simulink model "Zmixed_new"  (R2020b)
settings: Solver=FixedStepAuto  StartTime=0.0  StopTime=80000  FixedStep=1  RelTol=1e-3
values from neighbouring files (symbols this model uses):
  Inputp2 = data(1:IT,12)    [MainRun_step1__LoadData_and_DefineVaribles.m]
  InputT1 = data(1:IT,13)    [MainRun_step1__LoadData_and_DefineVaribles.m]
  InputWP = data(1:IT,66)    [MainRun_step1__LoadData_and_DefineVaribles.m]
  InputWT = data(1:IT,67)    [MainRun_step1__LoadData_and_DefineVaribles.m]
  Lp1 = data(1:IT,56)    [MainRun_step1__LoadData_and_DefineVaribles.m]
  Lp2 = data(1:IT,57)    [MainRun_step1__LoadData_and_DefineVaribles.m]
  T1 = data(1:IT,14)    [MainRun_step1__LoadData_and_DefineVaribles.m]
  Tamb = data(1:IT,55)    [MainRun_step1__LoadData_and_DefineVaribles.m]
  Tf1 = data(1:IT,16)    [MainRun_step1__LoadData_and_DefineVaribles.m]
  Tg1 = data(1:IT,53)    [MainRun_step1__LoadData_and_DefineVaribles.m]
  Tm = mean(data(1:IT,23:38),2)    [MainRun_step1__LoadData_and_DefineVaribles.m]
  WG = data(1:IT,51)    [MainRun_step1__LoadData_and_DefineVaribles.m]
  WR = data(1:IT,52)    [MainRun_step1__LoadData_and_DefineVaribles.m]
  Wtf = data(1:IT,15)    [MainRun_step1__LoadData_and_DefineVaribles.m]
  x = data(1:IT,49)    [MainRun_step1__LoadData_and_DefineVaribles.m]
  Zf = data(1:IT,50)    [MainRun_step1__LoadData_and_DefineVaribles.m]
undefined symbols (not defined in the file or in its folder): get_hs, precl, preclcp, precllamda, preclP, preclPP, preclT, refpropV
settings Model: Creator=Y7000  LastModifiedBy=admin
settings DataIOCC: ReturnWorkspaceOutputs=off
settings DebuggingCC: ArithmeticOperatorsInVariantConditions=warning
settings SFSimCC: CustomCodeUndefinedFunction=UseInterfaceOnly

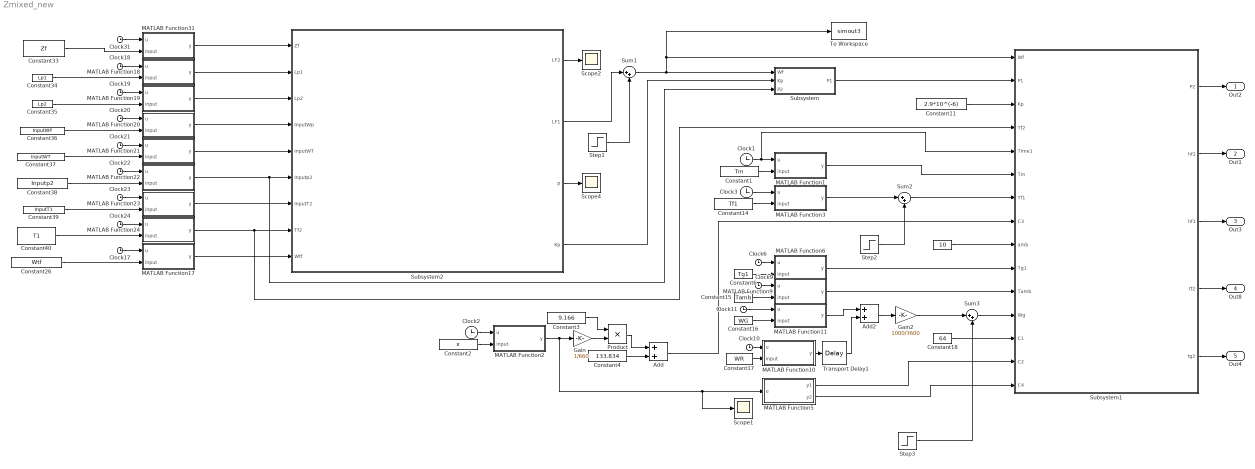
== system Zmixed_new ==
  " " : Constant  Value=10
  Add : Sum
  Add2 : Sum
  Clock{1..3,6,9..11,17..24,31} (16 alike) : Clock
  Constant1 : Constant  Value=Tm
  Constant11 : Constant  Value=2.9*10^(-6)
  Constant14 : Constant  Value=Tf1
  Constant15 : Constant  Value=Tamb
  Constant16 : Constant  Value=WG
  Constant17 : Constant  Value=WR
  Constant18 : Constant  Value=64
  Constant2 : Constant  Value=x
  Constant26 : Constant  Value=Wtf
  Constant3 : Constant  Value=9.166
  Constant33 : Constant  Value=Zf
  Constant34 : Constant  Value=Lp1
  Constant35 : Constant  Value=Lp2
  Constant36 : Constant  Value=InputWP
  Constant37 : Constant  Value=InputWT
  Constant38 : Constant  Value=Inputp2
  Constant39 : Constant  Value=InputT1
  Constant4 : Constant  Value=133.834
  Constant40 : Constant  Value=T1
  Constant6 : Constant  Value=Tg1
  Gain : Gain  Gain=1/660
  Gain2 : Gain  Gain=1000/3600
  MATLAB Function1 : MATLAB Function  TreatAsAtomicUnit=on
  MATLAB Function10 : MATLAB Function  TreatAsAtomicUnit=on
  MATLAB Function11 : MATLAB Function  TreatAsAtomicUnit=on
  MATLAB Function17 : MATLAB Function  TreatAsAtomicUnit=on
  MATLAB Function18 : MATLAB Function  TreatAsAtomicUnit=on
  MATLAB Function19 : MATLAB Function  TreatAsAtomicUnit=on
  MATLAB Function2 : MATLAB Function  TreatAsAtomicUnit=on
  MATLAB Function20 : MATLAB Function  TreatAsAtomicUnit=on
  MATLAB Function21 : MATLAB Function  TreatAsAtomicUnit=on
  MATLAB Function22 : MATLAB Function  TreatAsAtomicUnit=on
  MATLAB Function23 : MATLAB Function  TreatAsAtomicUnit=on
  MATLAB Function24 : MATLAB Function  TreatAsAtomicUnit=on
  MATLAB Function3 : MATLAB Function  TreatAsAtomicUnit=on
  MATLAB Function31 : MATLAB Function  TreatAsAtomicUnit=on
  MATLAB Function5 : MATLAB Function  TreatAsAtomicUnit=on
  MATLAB Function6 : MATLAB Function  TreatAsAtomicUnit=on
  MATLAB Function9 : MATLAB Function  TreatAsAtomicUnit=on
  Product : Product
  Scope1 : Scope
  Scope2 : Scope
  Scope4 : Scope
  Step1 : Step  After=0  SampleTime=1000
  Step2 : Step  After=0  SampleTime=1000
  Step3 : Step  After=0  SampleTime=1000
  Subsystem : Subsystem
  Subsystem1 : Subsystem
  Subsystem2 : Subsystem
  Sum1 : Sum  Inputs=|++
  Sum2 : Sum  Inputs=|++
  Sum3 : Sum  Inputs=|++
  To Workspace : ToWorkspace  VariableName=simout3  SaveFormat=Structure  SampleTime=-1
  Transport Delay1 : TransportDelay  DelayTime=37
  Out2 : Outport  VectorParamsAs1DForOutWhenUnconnected=off
  Out1 : Outport  Port=2  VectorParamsAs1DForOutWhenUnconnected=off
  Out3 : Outport  Port=3  VectorParamsAs1DForOutWhenUnconnected=off
  Out8 : Outport  Port=4  VectorParamsAs1DForOutWhenUnconnected=off
  Out4 : Outport  Port=5  VectorParamsAs1DForOutWhenUnconnected=off
  wires:
  Constant26/1 -> MATLAB Function17/2(input)
  Constant38/1 -> MATLAB Function22/2(input)
  MATLAB Function21/1(y) -> Subsystem2/5(InputWT)
  Subsystem1/3(hf1) -> Out3/1
  Constant40/1 -> MATLAB Function24/2(input)
  Constant11/1 -> Subsystem1/3(Kp)
  Subsystem1/2(hf2) -> Out1/1
  MATLAB Function20/1(y) -> Subsystem2/4(InputWp)
  MATLAB Function31/1(y) -> Subsystem2/1(Zf)
  Clock31/1 -> MATLAB Function31/1(u)
  Clock24/1 -> MATLAB Function24/1(u)
  MATLAB Function17/1(y) -> Subsystem2/9(Wtf)
  Clock18/1 -> MATLAB Function18/1(u)
  Constant34/1 -> MATLAB Function18/2(input)
  MATLAB Function23/1(y) -> Subsystem2/7(InputT2)
  Constant36/1 -> MATLAB Function20/2(input)
  Subsystem1/1(P2) -> Out2/1
  Clock22/1 -> MATLAB Function22/1(u)
  Constant39/1 -> MATLAB Function23/2(input)
  Constant37/1 -> MATLAB Function21/2(input)
  MATLAB Function19/1(y) -> Subsystem2/3(Lp2)
  Clock21/1 -> MATLAB Function21/1(u)
  Constant35/1 -> MATLAB Function19/2(input)
  MATLAB Function18/1(y) -> Subsystem2/2(Lp1)
  Constant33/1 -> MATLAB Function31/2(input)
  Constant14/1 -> MATLAB Function3/2(input)
  Subsystem2/1(LF2) -> Scope2/1
  Clock23/1 -> MATLAB Function23/1(u)
  Clock3/1 -> MATLAB Function3/1(u)
  Add/1 -> Subsystem1/8(C3)
  Subsystem2/4(Kp) -> Subsystem/2(Kp)
  Clock20/1 -> MATLAB Function20/1(u)
  Subsystem1/4(tf2) -> Out8/1
  Clock17/1 -> MATLAB Function17/1(u)
  Clock19/1 -> MATLAB Function19/1(u)
  Clock1/1 -> Subsystem1/5(Time1), MATLAB Function1/1(u)
  Constant1/1 -> MATLAB Function1/2(input)
  MATLAB Function1/1(y) -> Subsystem1/6(Tm)
  Subsystem2/3(p) -> Scope4/1
  MATLAB Function24/1(y) -> Subsystem1/4(Tf2), Subsystem2/8(Tf2)
  MATLAB Function22/1(y) -> Subsystem/3(P2), Subsystem2/6(Inputp2)
  Constant2/1 -> MATLAB Function2/2(input)
  Clock2/1 -> MATLAB Function2/1(u)
  Constant3/1 -> Product/1
  Product/1 -> Add/1
  Constant4/1 -> Add/2
  MATLAB Function2/1(y) -> MATLAB Function5/1(u), Scope1/1, Gain/1
  Gain/1 -> Product/2
  " "/1 -> Subsystem1/9(amb)
  Clock6/1 -> MATLAB Function6/1(u)
  Constant6/1 -> MATLAB Function6/2(input)
  MATLAB Function6/1(y) -> Subsystem1/10(Tg1)
  Constant15/1 -> MATLAB Function9/2(input)
  Clock9/1 -> MATLAB Function9/1(u)
  MATLAB Function9/1(y) -> Subsystem1/11(Tamb)
  Constant17/1 -> MATLAB Function10/2(input)
  Add2/1 -> Gain2/1
  Clock10/1 -> MATLAB Function10/1(u)
  MATLAB Function10/1(y) -> Transport Delay1/1
  Clock11/1 -> MATLAB Function11/1(u)
  Constant18/1 -> Subsystem1/13(C1)
  MATLAB Function5/1(y1) -> Subsystem1/14(C2)
  Constant16/1 -> MATLAB Function11/2(input)
  MATLAB Function11/1(y) -> Add2/1
  Transport Delay1/1 -> Add2/2
  MATLAB Function5/2(y2) -> Subsystem1/15(C4)
  Subsystem1/5(tg2) -> Out4/1
  Subsystem/1(P1) -> Subsystem1/2(P1)
  Step1/1 -> Sum1/2
  Subsystem2/2(LF1) -> Sum1/1
  Sum1/1 -> To Workspace/1, Subsystem1/1(Wf), Subsystem/1(Wf)
  Step2/1 -> Sum2/2
  MATLAB Function3/1(y) -> Sum2/1
  Sum2/1 -> Subsystem1/7(Tf1)
  Step3/1 -> Sum3/2
  Gain2/1 -> Sum3/1
  Sum3/1 -> Subsystem1/12(Wg)

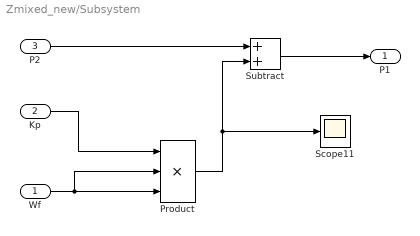
== system Zmixed_new/Subsystem ==
  Wf : Inport
  Kp : Inport  Port=2
  P2 : Inport  Port=3
  Product : Product  Inputs=3
  Scope11 : Scope
  Subtract : Sum
  P1 : Outport  VectorParamsAs1DForOutWhenUnconnected=off
  wires:
  Subtract/1 -> P1/1
  Wf/1 -> Product/2, Product/3
  Kp/1 -> Product/1
  P2/1 -> Subtract/1
  Product/1 -> Scope11/1, Subtract/2

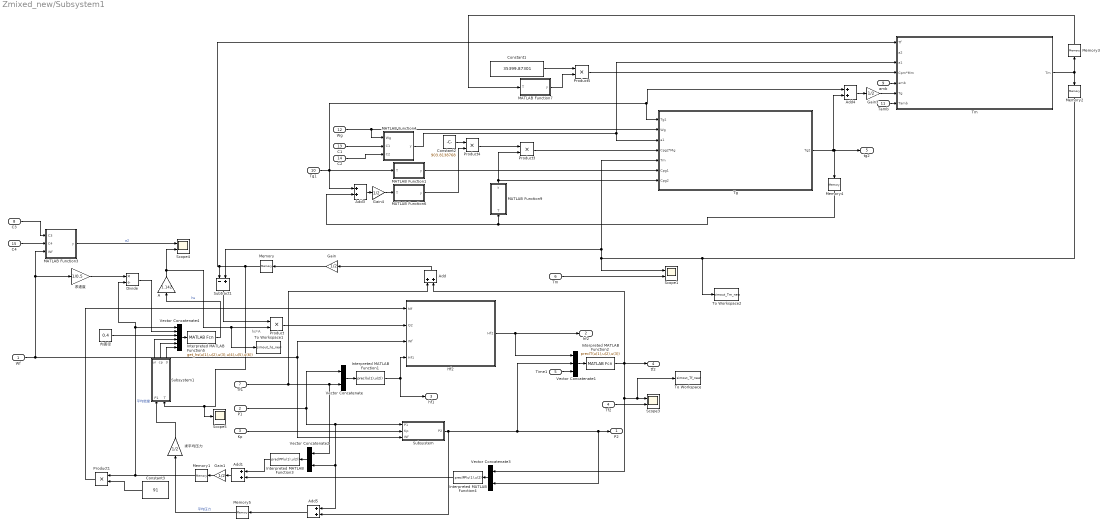
== system Zmixed_new/Subsystem1 ==
  note: hs*A
  Wf : Inport
  P1 : Inport  Port=2
  Kp : Inport  Port=3
  Tf2 : Inport  Port=4
  Time1 : Inport  Port=5
  Tm : Inport  Port=6
  Tf1 : Inport  Port=7
  C3 : Inport  Port=8
  amb : Inport  Port=9
  Tg1 : Inport  Port=10
  Tamb : Inport  Port=11
  Wg : Inport  Port=12
  C1 : Inport  Port=13
  C2 : Inport  Port=14
  C4 : Inport  Port=15
  A : Gain  Gain=1.142
  Add{,1,3..5} (5 alike) : Sum
  Constant1 : Constant  Value=35399.87301
  Constant2 : Constant  Value=903.8138768
  Constant3 : Constant  Value=91
  Divide : Product  Inputs=*/
  Gain{,1,3..4} (4 alike) : Gain  Gain=1/2
  Hf2 : Subsystem
  Interpreted MATLAB Function1 : MATLABFcn  MATLABFcn=precl(u(1),u(2))
  Interpreted MATLAB Function2 : MATLABFcn  MATLABFcn=preclT(u(1),u(2),u(3))
  Interpreted MATLAB Function3 : MATLABFcn  MATLABFcn=preclPP(u(1),u(2))
  Interpreted MATLAB Function4 : MATLABFcn  MATLABFcn=preclPP(u(1),u(2))
  Interpreted MATLAB Function5 : MATLABFcn  MATLABFcn=get_hs(u(1),u(2),u(3),u(4),u(5),u(6))
  MATLAB Function1 : MATLAB Function  TreatAsAtomicUnit=on
  MATLAB Function3 : MATLAB Function  TreatAsAtomicUnit=on
  MATLAB Function4 : MATLAB Function  TreatAsAtomicUnit=on
  MATLAB Function6 : MATLAB Function  TreatAsAtomicUnit=on
  MATLAB Function7 : MATLAB Function  TreatAsAtomicUnit=on
  MATLAB Function9 : MATLAB Function  TreatAsAtomicUnit=on
  Memory : Memory  InitialCondition=450
  Memory1 : Memory  InitialCondition=52
  Memory2 : Memory
  Memory3 : Memory
  Memory4 : Memory
  Memory5 : Memory  InitialCondition=52
  Product{,1,3..5} (5 alike) : Product
  Scope1 : Scope  NumInputPorts=2
  Scope3 : Scope  NumInputPorts=2
  Scope4 : Scope  NumInputPorts=2
  Scope5 : Scope
  Subsystem : Subsystem
  Subsystem1 : Subsystem
  Subtract1 : Sum  Inputs=-+
  Tg : Subsystem
  "Tm " : Subsystem
  To Workspace : ToWorkspace  VariableName=simout_Tf_new  SaveFormat=Structure  SampleTime=-1
  To Workspace1 : ToWorkspace  VariableName=simout_hs_new  SaveFormat=Structure  SampleTime=-1
  To Workspace2 : ToWorkspace  VariableName=simout_Tm_new  SaveFormat=Structure  SampleTime=-1
  Vector Concatenate : Concatenate
  Vector Concatenate1 : Concatenate  NumInputs=3
  Vector Concatenate2 : Concatenate
  Vector Concatenate3 : Concatenate
  Vector Concatenate4 : Concatenate  NumInputs=6
  内直径 : Constant  Value=0.4
  求平均压力 : Gain  Gain=1/2
  求速度 : Gain  Gain=1/0.5
  P2 : Outport  VectorParamsAs1DForOutWhenUnconnected=off
  hf2 : Outport  Port=2  VectorParamsAs1DForOutWhenUnconnected=off
  hf1 : Outport  Port=3  VectorParamsAs1DForOutWhenUnconnected=off
  tf2 : Outport  Port=4  VectorParamsAs1DForOutWhenUnconnected=off
  tg2 : Outport  Port=5  VectorParamsAs1DForOutWhenUnconnected=off
  wires:
  C3/1 -> MATLAB Function3/1(C3)
  Add/1 -> Gain/1
  Kp/1 -> Subsystem/2(Kp)
  Vector Concatenate/1 -> Interpreted MATLAB Function1/1
  Interpreted MATLAB Function1/1 -> Hf2/4(Hf1), hf1/1
  Product1/1 -> Hf2/1(Mf)
  Product/1 -> Hf2/2(Q2)
  Hf2/1(Hf2) -> Vector Concatenate1/1, hf2/1
  Vector Concatenate1/1 -> Interpreted MATLAB Function2/1
  Time1/1 -> Vector Concatenate1/3
  Wf/1 -> Hf2/3(Wf), Subsystem/3(Wf), 求速度/1, MATLAB Function3/3(Wf)
  Interpreted MATLAB Function2/1 -> Vector Concatenate3/1, Scope3/1, To Workspace/1, tf2/1, Add/2
  Gain/1 -> Memory/1
  Memory/1 -> "Tm "/1(Tf), Subtract1/1, Scope5/1, Subsystem1/2(T)
  Subtract1/1 -> Product/1
  Tf1/1 -> Vector Concatenate/2, Vector Concatenate2/1, Add/1
  P1/1 -> Add5/1, Vector Concatenate2/2, Subsystem/1(P1), Vector Concatenate/1
  Vector Concatenate2/1 -> Interpreted MATLAB Function3/1
  Vector Concatenate3/1 -> Interpreted MATLAB Function4/1
  Subsystem/1(P2) -> P2/1, Vector Concatenate3/2, Vector Concatenate1/2, Add5/2
  Tf2/1 -> Scope3/2
  Interpreted MATLAB Function4/1 -> Add1/2
  Interpreted MATLAB Function3/1 -> Add1/1
  Add1/1 -> Gain1/1
  Constant3/1 -> Product1/2
  Gain1/1 -> Memory1/1
  Memory1/1 -> Divide/2, Vector Concatenate4/1, Product1/1  "平均密度"
  C4/1 -> MATLAB Function3/2(C4)
  Gain3/1 -> "Tm "/6(Tg)
  Product3/1 -> Tg/4(Cpg2*Mg)
  amb/1 -> "Tm "/5(amb)
  Constant2/1 -> Product4/1
  MATLAB Function4/1(y) -> Tg/3(a1), "Tm "/3(a1)
  Tg1/1 -> Add3/1, Add4/1, Tg/1(Tg1), MATLAB Function1/1(T)
  MATLAB Function9/1(y) -> Product3/2, Tg/7(Cpg2)
  Product5/1 -> "Tm "/4(Cpm*Mm)
  Add4/1 -> Gain3/1
  Wg/1 -> MATLAB Function4/1(Wg), Tg/2(Wg)
  Tamb/1 -> "Tm "/7(Tamb)
  C2/1 -> MATLAB Function4/3(C2)
  MATLAB Function6/1(y) -> Product4/2
  MATLAB Function1/1(y) -> Tg/6(Cpg1)
  Add3/1 -> Gain4/1
  MATLAB Function7/1(y) -> Product5/2
  C1/1 -> MATLAB Function4/2(C1)
  Tg/1(Tg2) -> tg2/1, Memory4/1, Add4/2
  Gain4/1 -> MATLAB Function6/1(T)
  Constant1/1 -> Product5/1
  "Tm "/1(Tm) -> Memory2/1, Memory3/1
  Product4/1 -> Product3/1
  Memory4/1 -> MATLAB Function9/1(T), Add3/2
  Memory3/1 -> MATLAB Function7/1(T)
  Memory2/1 -> To Workspace2/1, Tg/5(Tm), Subtract1/2, Scope1/1
  MATLAB Function3/1(y) -> Scope4/1  "a2"
  求速度/1 -> Divide/1
  Vector Concatenate4/1 -> Interpreted MATLAB Function5/1
  内直径/1 -> Vector Concatenate4/3
  Add5/1 -> Memory5/1
  求平均压力/1 -> Subsystem1/1(P1)
  Subsystem1/1(ur) -> Vector Concatenate4/4
  Subsystem1/2(cp) -> Vector Concatenate4/5
  Memory5/1 -> 求平均压力/1  "平均压力"
  Interpreted MATLAB Function5/1 -> A/1  "hs"
  Subsystem1/3(lamda) -> Vector Concatenate4/6
  Divide/1 -> Vector Concatenate4/2
  A/1 -> To Workspace1/1, Product/2, Scope4/2
  Tm/1 -> Scope1/2

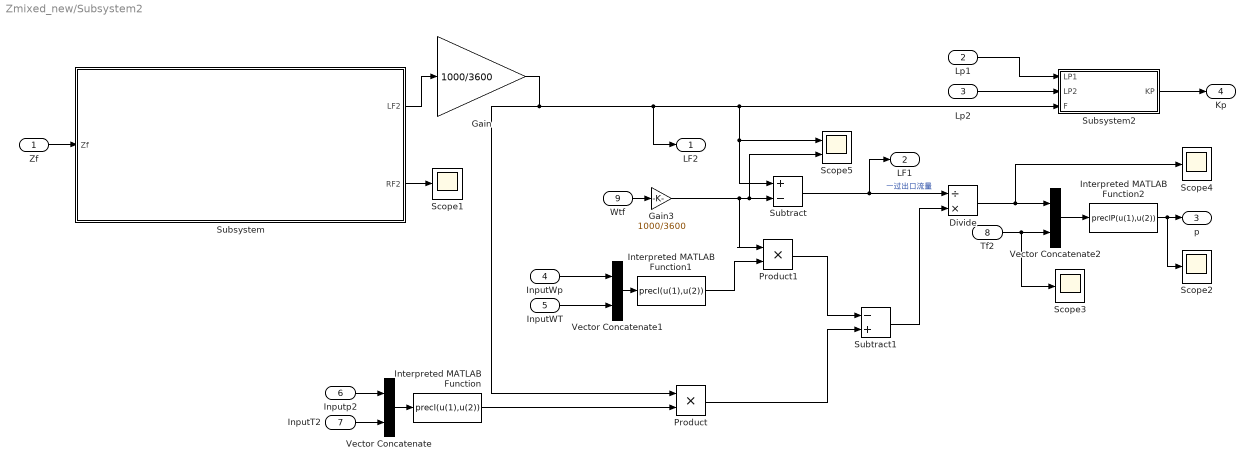
== system Zmixed_new/Subsystem2 ==
  Zf : Inport
  Lp1 : Inport  Port=2
  Lp2 : Inport  Port=3
  InputWp : Inport  Port=4
  InputWT : Inport  Port=5
  Inputp2 : Inport  Port=6
  InputT2 : Inport  Port=7
  Tf2 : Inport  Port=8
  Wtf : Inport  Port=9
  Divide : Product  Inputs=/*
  Gain : Gain  Gain=1000/3600
  Gain3 : Gain  Gain=1000/3600
  Interpreted MATLAB Function : MATLABFcn  MATLABFcn=precl(u(1),u(2))
  Interpreted MATLAB Function1 : MATLABFcn  MATLABFcn=precl(u(1),u(2))
  Interpreted MATLAB Function2 : MATLABFcn  MATLABFcn=preclP(u(1),u(2))
  Product : Product
  Product1 : Product
  Scope{1..4} (4 alike) : Scope
  Scope5 : Scope  NumInputPorts=2
  Subsystem : Subsystem
  Subsystem2 : Subsystem
  Subtract : Sum  Inputs=+-
  Subtract1 : Sum  Inputs=-+
  Vector Concatenate : Concatenate
  Vector Concatenate1 : Concatenate
  Vector Concatenate2 : Concatenate
  LF2 : Outport  VectorParamsAs1DForOutWhenUnconnected=off
  LF1 : Outport  Port=2  VectorParamsAs1DForOutWhenUnconnected=off
  p : Outport  Port=3  VectorParamsAs1DForOutWhenUnconnected=off
  Kp : Outport  Port=4  VectorParamsAs1DForOutWhenUnconnected=off
  wires:
  Wtf/1 -> Gain3/1
  Subsystem2/1(KP) -> Kp/1
  Interpreted MATLAB Function1/1 -> Product1/2
  Interpreted MATLAB Function/1 -> Product/2
  Product1/1 -> Subtract1/1
  Product/1 -> Subtract1/2
  Subtract/1 -> LF1/1, Divide/1  "一过出口流量"
  Subtract1/1 -> Divide/2
  Divide/1 -> Scope4/1, Vector Concatenate2/1
  Subsystem/2(RF2) -> Scope1/1
  Zf/1 -> Subsystem/1(Zf)
  Lp1/1 -> Subsystem2/1(LP1)
  Lp2/1 -> Subsystem2/2(LP2)
  InputWp/1 -> Vector Concatenate1/1
  InputWT/1 -> Vector Concatenate1/2
  Inputp2/1 -> Vector Concatenate/1
  Tf2/1 -> Scope3/1, Vector Concatenate2/2
  Vector Concatenate/1 -> Interpreted MATLAB Function/1
  InputT2/1 -> Vector Concatenate/2
  Vector Concatenate1/1 -> Interpreted MATLAB Function1/1
  Vector Concatenate2/1 -> Interpreted MATLAB Function2/1
  Interpreted MATLAB Function2/1 -> Scope2/1, p/1
  Subsystem/1(LF2) -> Gain/1
  Gain/1 -> Product/1, Subsystem2/3(F), Scope5/1, Subtract/1, LF2/1
  Gain3/1 -> Product1/1, Scope5/2, Subtract/2

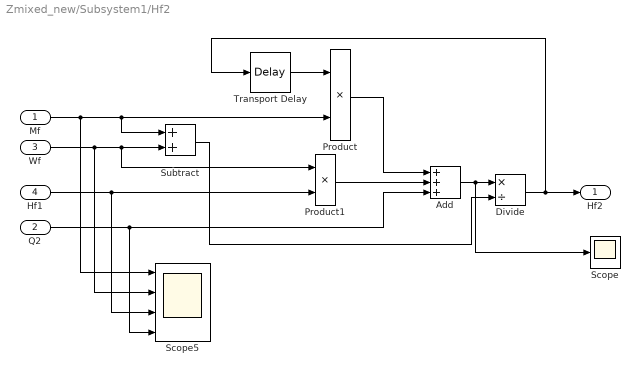
== system Zmixed_new/Subsystem1/Hf2 ==
  Mf : Inport
  Q2 : Inport  Port=2
  Wf : Inport  Port=3
  Hf1 : Inport  Port=4
  Add : Sum  Inputs=+++
  Divide : Product  Inputs=*/
  Product : Product
  Product1 : Product
  Scope : Scope
  Scope5 : Scope  NumInputPorts=4
  Subtract : Sum
  Transport Delay : TransportDelay
  Hf2 : Outport  VectorParamsAs1DForOutWhenUnconnected=off
  wires:
  Q2/1 -> Scope5/4, Add/3
  Subtract/1 -> Divide/2
  Hf1/1 -> Scope5/3, Product1/2
  Add/1 -> Scope/1, Divide/1
  Product1/1 -> Add/2
  Divide/1 -> Hf2/1, Transport Delay/1
  Product/1 -> Add/1
  Mf/1 -> Scope5/1, Subtract/1, Product/2
  Transport Delay/1 -> Product/1
  Wf/1 -> Scope5/2, Product1/1, Subtract/2

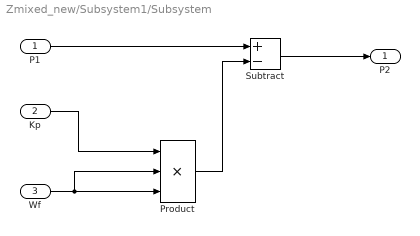
== system Zmixed_new/Subsystem1/Subsystem ==
  P1 : Inport
  Kp : Inport  Port=2
  Wf : Inport  Port=3
  Product : Product  Inputs=3
  Subtract : Sum  Inputs=+-
  P2 : Outport  VectorParamsAs1DForOutWhenUnconnected=off
  wires:
  Subtract/1 -> P2/1
  Wf/1 -> Product/2, Product/3
  Kp/1 -> Product/1
  P1/1 -> Subtract/1
  Product/1 -> Subtract/2

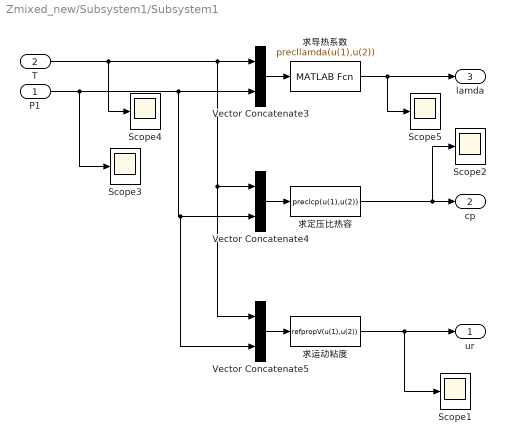
== system Zmixed_new/Subsystem1/Subsystem1 ==
  P1 : Inport
  T : Inport  Port=2
  Scope{1..5} (5 alike) : Scope
  Vector Concatenate3 : Concatenate
  Vector Concatenate4 : Concatenate
  Vector Concatenate5 : Concatenate
  求定压比热容 : MATLABFcn  MATLABFcn=preclcp(u(1),u(2))
  求导热系数 : MATLABFcn  MATLABFcn=precllamda(u(1),u(2))
  求运动粘度 : MATLABFcn  MATLABFcn=refpropV(u(1),u(2))
  ur : Outport  VectorParamsAs1DForOutWhenUnconnected=off
  cp : Outport  Port=2  VectorParamsAs1DForOutWhenUnconnected=off
  lamda : Outport  Port=3  VectorParamsAs1DForOutWhenUnconnected=off
  wires:
  Vector Concatenate5/1 -> 求运动粘度/1
  Vector Concatenate4/1 -> 求定压比热容/1
  Vector Concatenate3/1 -> 求导热系数/1
  T/1 -> Scope4/1, Vector Concatenate5/1, Vector Concatenate4/1, Vector Concatenate3/1
  求运动粘度/1 -> Scope1/1, ur/1
  求定压比热容/1 -> Scope2/1, cp/1
  求导热系数/1 -> Scope5/1, lamda/1
  P1/1 -> Scope3/1, Vector Concatenate5/2, Vector Concatenate4/2, Vector Concatenate3/2

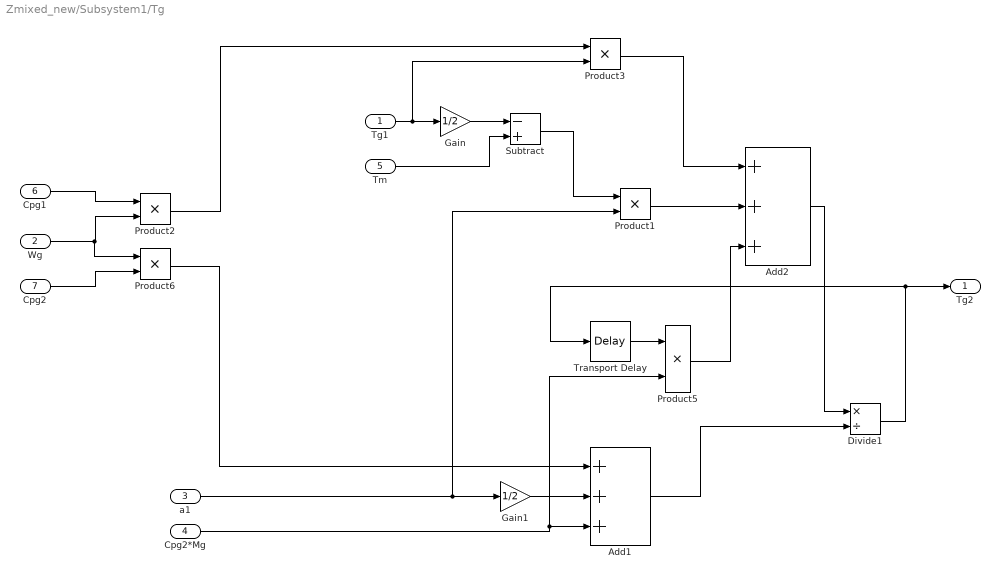
== system Zmixed_new/Subsystem1/Tg ==
  Tg1 : Inport
  Wg : Inport  Port=2
  a1 : Inport  Port=3
  Cpg2*Mg : Inport  Port=4
  Tm : Inport  Port=5
  Cpg1 : Inport  Port=6
  Cpg2 : Inport  Port=7
  Add1 : Sum  Inputs=+++
  Add2 : Sum  Inputs=+++
  Divide1 : Product  Inputs=*/
  Gain : Gain  Gain=1/2
  Gain1 : Gain  Gain=1/2
  Product{1..3,5..6} (5 alike) : Product
  Subtract : Sum  Inputs=-+
  Transport Delay : TransportDelay
  Tg2 : Outport  VectorParamsAs1DForOutWhenUnconnected=off
  wires:
  Cpg2*Mg/1 -> Add1/3, Product5/2
  a1/1 -> Product1/2, Gain1/1
  Tm/1 -> Subtract/2
  Divide1/1 -> Tg2/1, Transport Delay/1
  Add1/1 -> Divide1/2
  Transport Delay/1 -> Product5/1
  Product3/1 -> Add2/1
  Product1/1 -> Add2/2
  Product5/1 -> Add2/3
  Add2/1 -> Divide1/1
  Cpg1/1 -> Product2/1
  Wg/1 -> Product6/1, Product2/2
  Cpg2/1 -> Product6/2
  Product6/1 -> Add1/1
  Product2/1 -> Product3/1
  Tg1/1 -> Product3/2, Gain/1
  Gain/1 -> Subtract/1
  Subtract/1 -> Product1/1
  Gain1/1 -> Add1/2

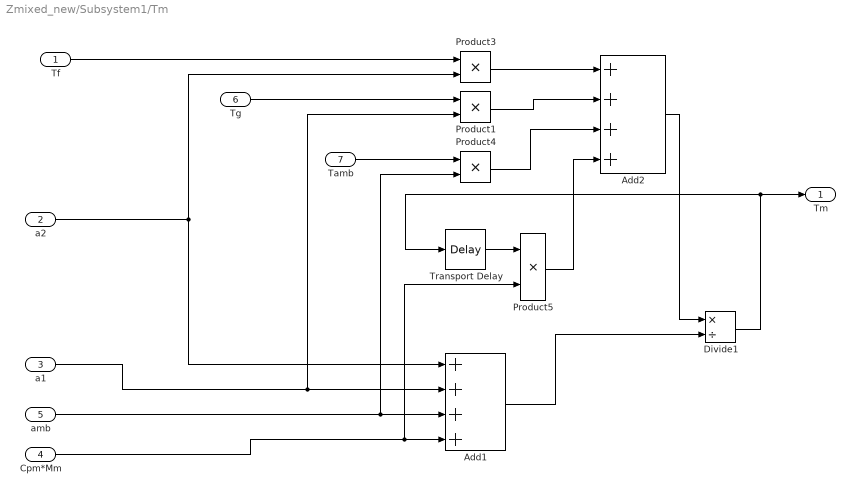
== system Zmixed_new/Subsystem1/Tm  ==
  Tf : Inport
  a2 : Inport  Port=2
  a1 : Inport  Port=3
  Cpm*Mm : Inport  Port=4
  amb : Inport  Port=5
  Tg : Inport  Port=6
  Tamb : Inport  Port=7
  Add1 : Sum  Inputs=++++
  Add2 : Sum  Inputs=++++
  Divide1 : Product  Inputs=*/
  Product{1,3..5} (4 alike) : Product
  Transport Delay : TransportDelay
  Tm : Outport  VectorParamsAs1DForOutWhenUnconnected=off
  wires:
  Tf/1 -> Product3/1
  amb/1 -> Product4/2, Add1/3
  Cpm*Mm/1 -> Product5/2, Add1/4
  a1/1 -> Product1/2, Add1/2
  a2/1 -> Product3/2, Add1/1
  Tg/1 -> Product1/1
  Tamb/1 -> Product4/1
  Divide1/1 -> Tm/1, Transport Delay/1
  Add1/1 -> Divide1/2
  Transport Delay/1 -> Product5/1
  Product3/1 -> Add2/1
  Product1/1 -> Add2/2
  Product4/1 -> Add2/3
  Product5/1 -> Add2/4
  Add2/1 -> Divide1/1

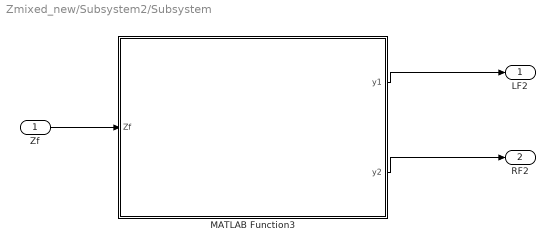
== system Zmixed_new/Subsystem2/Subsystem ==
  Zf : Inport
  MATLAB Function3 : MATLAB Function  TreatAsAtomicUnit=on
  LF2 : Outport  VectorParamsAs1DForOutWhenUnconnected=off
  RF2 : Outport  Port=2  VectorParamsAs1DForOutWhenUnconnected=off
  wires:
  Zf/1 -> MATLAB Function3/1(Zf)
  MATLAB Function3/2(y2) -> RF2/1
  MATLAB Function3/1(y1) -> LF2/1

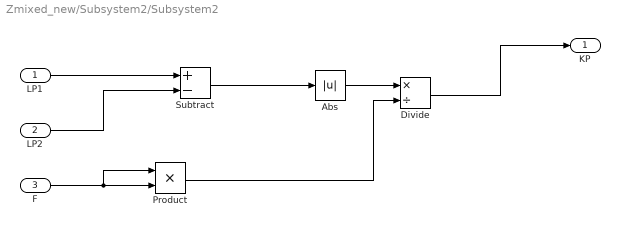
== system Zmixed_new/Subsystem2/Subsystem2 ==
  LP1 : Inport
  LP2 : Inport  Port=2
  F : Inport  Port=3
  Abs : Abs
  Divide : Product  Inputs=*/
  Product : Product
  Subtract : Sum  Inputs=+-
  KP : Outport  VectorParamsAs1DForOutWhenUnconnected=off
  wires:
  LP1/1 -> Subtract/1
  LP2/1 -> Subtract/2
  Subtract/1 -> Abs/1
  Abs/1 -> Divide/1
  F/1 -> Product/1, Product/2
  Product/1 -> Divide/2
  Divide/1 -> KP/1

== matlab function Zmixed_new/Subsystem1/MATLAB Function6 ==
  data: T input; y output
function y = fcn(T)
n=400:100:1200;
m=[0.52,0.45,0.4,0.3,0.28,0.275,0.225,0.215,0.2];
y =interp1(n,m,T,'spline');

== matlab function Zmixed_new/Subsystem1/MATLAB Function7 ==
  data: T input; y output
function y = fcn(T)
n=400:100:600;
m=[0.528,0.551,0.581];
y =interp1(n,m,T,'spline');

== matlab function Zmixed_new/MATLAB Function17 ==
  data: u input; y output; input input
function y = fcn(u,input)
 c=fix(u/1);
if u==0 ||c==0
    y=input(1);
else
    y=input(c);
% y=U3(u);
end

== matlab function Zmixed_new/MATLAB Function18 ==
  data: u input; y output; input input
function y = fcn(u,input)
 c=fix(u/1);
if u==0 ||c==0
    y=input(1);
else
    y=input(c);
% y=U3(u);
end

== matlab function Zmixed_new/MATLAB Function19 ==
  data: u input; y output; input input
function y = fcn(u,input)
 c=fix(u/1);
if u==0 ||c==0
    y=input(1);
else
    y=input(c);
% y=U3(u);
end

== matlab function Zmixed_new/MATLAB Function1 ==
  data: u input; y output; input input
function y = fcn(u,input)
 c=fix(u/1);
if u==0 ||c==0
    y=input(1);
else
    y=input(c);
% y=U3(u);
end

== matlab function Zmixed_new/MATLAB Function20 ==
  data: u input; y output; input input
function y = fcn(u,input)
 c=fix(u/1);
if u==0 ||c==0
    y=input(1);
else
    y=input(c);
% y=U3(u);
end

== matlab function Zmixed_new/MATLAB Function21 ==
  data: u input; y output; input input
function y = fcn(u,input)
 c=fix(u/1);
if u==0 ||c==0
    y=input(1);
else
    y=input(c);
% y=U3(u);
end

== matlab function Zmixed_new/MATLAB Function22 ==
  data: u input; y output; input input
function y = fcn(u,input)
 c=fix(u/1);
if u==0 ||c==0
    y=input(1);
else
    y=input(c);
% y=U3(u);
end

== matlab function Zmixed_new/MATLAB Function23 ==
  data: u input; y output; input input
function y = fcn(u,input)
 c=fix(u/1);
if u==0 ||c==0
    y=input(1);
else
    y=input(c);
% y=U3(u);
end

== matlab function Zmixed_new/MATLAB Function24 ==
  data: u input; y output; input input
function y = fcn(u,input)
 c=fix(u/1);
if u==0 ||c==0
    y=input(1);
else
    y=input(c);
% y=U3(u);
end

== matlab function Zmixed_new/Subsystem1/MATLAB Function9 ==
  data: T input; y output
function y = fcn(T)
n=400:100:1200;
m=[1.15,1.2,1.23,1.25,1.275,1.285,1.3,1.32,1.33];
y =interp1(n,m,T,'spline');

== matlab function Zmixed_new/MATLAB Function31 ==
  data: u input; y output; input input
function y = fcn(u,input)
 c=fix(u/1);
if u==0 ||c==0
    y=input(1);
else
    y=input(c);
% y=U3(u);
end

== matlab function Zmixed_new/Subsystem2/Subsystem/MATLAB Function3 ==
  data: Zf input; y1 output; y2 output
function [y1,y2]= fcn(Zf)

    y1=Zf*1/2;
    y2=Zf*1/2;

== matlab function Zmixed_new/MATLAB Function2 ==
  data: u input; y output; input input
function y = fcn(u,input)
 c=fix(u/1);
if u==0 ||c==0
    y=input(1);
else
    y=input(c);
% y=U3(u);
end

== matlab function Zmixed_new/Subsystem1/MATLAB Function3 ==
  data: C3 input; C4 input; Wf input; y output
function y = fcn(C3,C4,Wf)

y = C3+C4*Wf.^0.8;

== matlab function Zmixed_new/MATLAB Function5 ==
  data: u input; y1 output; y2 output
function [y1,y2]= fcn(u)
if u>550
    y1=2;
    y2=37;
else
    if u>500
        y1=2;
        y2=34;
    else
         if u>300
           y1=5;
           y2=32;
         else
           y1=5;
           y2=10;
         end
    end
end

== matlab function Zmixed_new/MATLAB Function3 ==
  data: u input; y output; input input
function y = fcn(u,input)
 c=fix(u/1);
if u==0 ||c==0
    y=input(1);
else
    y=input(c);
% y=U3(u);
end

== matlab function Zmixed_new/MATLAB Function6 ==
  data: u input; y output; input input
function y = fcn(u,input)
 c=fix(u/1);
if u==0 ||c==0
    y=input(1);
else
    y=input(c);
% y=U3(u);
end

== matlab function Zmixed_new/MATLAB Function9 ==
  data: u input; y output; input input
function y = fcn(u,input)
 c=fix(u/1);
if u==0 ||c==0
    y=input(1);
else
    y=input(c);
% y=U3(u);
end

== matlab function Zmixed_new/MATLAB Function10 ==
  data: u input; y output; input input
function y = fcn(u,input)
 c=fix(u/1);
if u==0 ||c==0
    y=input(1);
else
    y=input(c);
% y=U3(u);
end

== matlab function Zmixed_new/MATLAB Function11 ==
  data: u input; y output; input input
function y = fcn(u,input)
 c=fix(u/1);
if u==0 ||c==0
    y=input(1);
else
    y=input(c);
% y=U3(u);
end

== matlab function Zmixed_new/Subsystem1/MATLAB Function1 ==
  data: T input; y output
function y = fcn(T)
n=400:100:1200;
m=[1.15,1.2,1.23,1.25,1.275,1.285,1.3,1.32,1.33];
y =interp1(n,m,T,'spline');

== matlab function Zmixed_new/Subsystem1/MATLAB Function4 ==
  data: Wg input; C1 input; y output; C2 input
function y = fcn(Wg,C1,C2)

y = C1+C2*Wg.^0.68;
